simulink model "PositionObserver"  (R2020b)
settings: Solver=FixedStepDiscrete  StartTime=0.0  StopTime=100  RelTol=1e-3
values from neighbouring files (symbols this model uses):
  Ki_Iab_EMFobs = 1600.0    [MotorControl.sldd]
  Kp_Iab_EMFobs = 0.255    [MotorControl.sldd]
  Ts = 250.0e-06    (= 0.00025)    [MotorControlLibData.m]    (also in local_pmsm_torque_control_data.m = 5e-06)
undefined symbols (not defined in the file or in its folder): CuttOffFreq_c, EMFobsLdGain, EMFobsRS, MaxBckEMFVol_sat_neg, MaxBckEMFVol_sat_pos, TsIntern
libraries: pid_lib x2
settings Model: DataDictionary=MotorControl.sldd  Creator=unix  LastModifiedBy=unix
settings SolverCC: AutoInsertRateTranBlk=on
settings DataIOCC: SaveOutput=off  SaveTime=off
settings OptimizationCC: DefaultParameterBehavior=Inlined  EnhancedBackFolding=on  PassReuseOutputArgsAs=Individual arguments  ZeroExternalMemoryAtStartup=off  ZeroInternalMemoryAtStartup=off  OptimizeBlockOrder=speed  DifferentSizesBufferReuse=on  OptimizationCustomize=off  EfficientTunableParamExpr=on
settings DebuggingCC: SignalInfNanChecking=warning  SignalRangeChecking=warning  CheckMatrixSingularityMsg=warning  IntegerOverflowMsg=error  ParameterOverflowMsg=warning  ParameterUnderflowMsg=warning  ParameterPrecisionLossMsg=none  ParameterTunabilityLossMsg=error  UnderSpecifiedDataTypeMsg=warning  IntegerSaturationMsg=error
settings ModelReferenceCC: ModelReferenceNumInstancesAllowed=Single
settings SFSimCC: MATLABDynamicMemAlloc=off
settings RTWCC: Description=Embedded Coder  SystemTargetFile=ert.tlc  GenCodeOnly=on  TemplateMakefile=ert_default_tmf  GenerateReport=on  IncludeHyperlinkInReport=on  LaunchReport=on  GenerateTraceInfo=on  GenerateTraceReport=on  GenerateTraceReportSl=on  GenerateTraceReportSf=on  GenerateTraceReportEml=on
settings CodeAppCC: ForceParamTrailComments=on  IgnoreCustomStorageClasses=off  OperatorAnnotations=on  SimulinkDataObjDesc=on  SFDataObjDesc=on  InsertBlockDesc=on
settings ERTTargetCC: TargetLangStandard=C99 (ISO)  GenerateSampleERTMain=on  GenerateASAP2=on  InlinedParameterPlacement=NonHierarchical  ERTCustomFileTemplate=example_file_process.tlc

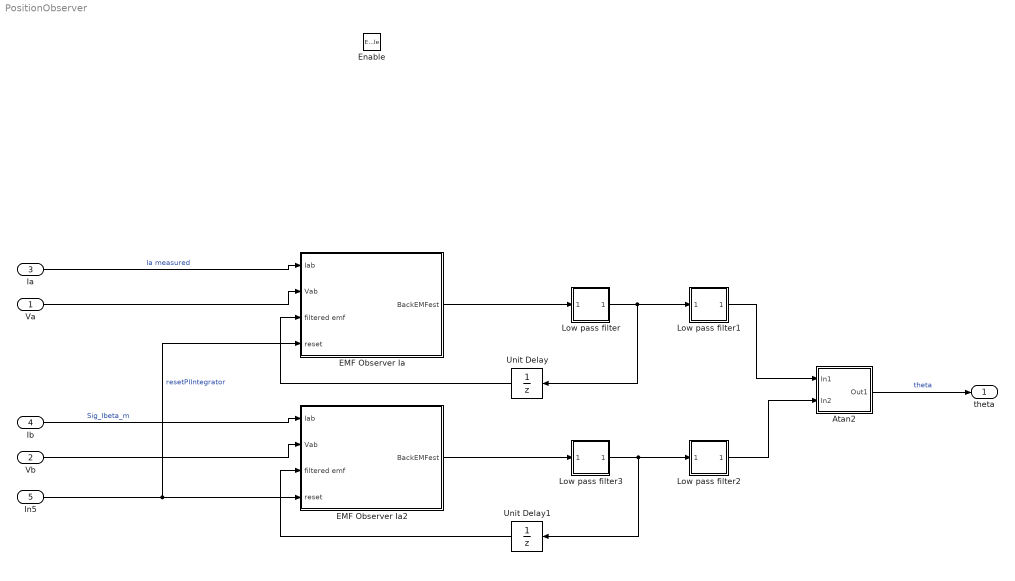
== system PositionObserver ==
  Va : Inport  OutDataTypeStr=fixdt(1,16,8)  PortDimensions=1  SampleTime=[0.00025000000000000001,0]
  Vb : Inport  Port=2  OutDataTypeStr=fixdt(1,16,8)  PortDimensions=1  SampleTime=[0.00025000000000000001,0]
  Ia : Inport  Port=3  OutDataTypeStr=fixdt(1,16,8)  PortDimensions=1  SampleTime=[0.00025000000000000001,0]
  Ib : Inport  Port=4  OutDataTypeStr=fixdt(1,16,8)  PortDimensions=1  SampleTime=[0.00025000000000000001,0]
  In5 : Inport  Port=5  OutDataTypeStr=boolean  PortDimensions=1  SampleTime=[0.00025000000000000001,0]
  Enable : EnablePort  StatesWhenEnabling=reset  SampleTime=[0.00025000000000000001,0]  OutDataTypeStr=boolean
  Atan2 : Subsystem
  EMF Observer Ia : Subsystem  mask{Rs=EMFobsRS, Ld=EMFobsLdGain, P=Kp_Iab_EMFobs, I=Ki_Iab_EMFobs}
      mask prompts: Rs "Resistance"; Ld "Inductance"; P "Simulink:masks:ProportionalP_MP"; I "Simulink:masks:IntegralI_MP"
      mask TypeOptions Rs: DC Motor Model/Resistance/Gain
      mask TypeOptions Ld: DC Motor Model/Inductance/Gain
      mask TypeOptions P: PID Controller/P
      mask TypeOptions I: PID Controller/I
      mask DialogControl Container6 Prompt: PI Controller
      mask DialogControl P Prompt: Proportional (P):
      mask DialogControl I Prompt: Integral (I):
  EMF Observer Ia2 : Subsystem  mask{Rs=EMFobsRS, Ld=EMFobsLdGain, P=Kp_Iab_EMFobs, I=Ki_Iab_EMFobs}
      mask prompts: Rs "Resistance"; Ld "Inductance"; P "Simulink:masks:ProportionalP_MP"; I "Simulink:masks:IntegralI_MP"
      mask TypeOptions Rs: DC Motor Model/Resistance/Gain
      mask TypeOptions Ld: DC Motor Model/Inductance/Gain
      mask TypeOptions P: PID Controller/P
      mask TypeOptions I: PID Controller/I
      mask DialogControl Container6 Prompt: PI Controller
      mask DialogControl P Prompt: Proportional (P):
      mask DialogControl I Prompt: Integral (I):
  Low pass filter : Subsystem  mask{Value=CuttOffFreq_c, Gain=250e-6}
      mask prompts: Value "CuttOff Freq."; Gain "Time interval"
      settings: AttributesFormatString=Integration constant %<Gain>
      mask TypeOptions Value: Constant/Value
      mask TypeOptions Gain: Gain/Gain
  Low pass filter1 : Subsystem  mask{Value=CuttOffFreq_c, Gain=250e-6}
      mask prompts: Value "CuttOff Freq."; Gain "Time interval"
      settings: AttributesFormatString=Integration constant %<Gain>
      mask TypeOptions Value: Constant/Value
      mask TypeOptions Gain: Gain/Gain
  Low pass filter2 : Subsystem  mask{Value=CuttOffFreq_c, Gain=250e-6}
      mask prompts: Value "CuttOff Freq."; Gain "Time interval"
      settings: AttributesFormatString=Integration constant %<Gain>
      mask TypeOptions Value: Constant/Value
      mask TypeOptions Gain: Gain/Gain
  Low pass filter3 : Subsystem  mask{Value=CuttOffFreq_c, Gain=250e-6}
      mask prompts: Value "CuttOff Freq."; Gain "Time interval"
      settings: AttributesFormatString=Integration constant %<Gain>
      mask TypeOptions Value: Constant/Value
      mask TypeOptions Gain: Gain/Gain
  Unit Delay : UnitDelay  SampleTime=-1  HasFrameUpgradeWarning=on
  Unit Delay1 : UnitDelay  SampleTime=-1  HasFrameUpgradeWarning=on
  theta : Outport  OutDataTypeStr=fixdt(1,16,8)  PortDimensions=1  SampleTime=[0.00025000000000000001,0]
  wires:
  Atan2/1(Out1) -> theta/1  "theta"
  Va/1 -> EMF Observer Ia/2(Vab)
  Ia/1 -> EMF Observer Ia/1(Iab)  "Ia measured"
  Vb/1 -> EMF Observer Ia2/2(Vab)
  Ib/1 -> EMF Observer Ia2/1(Iab)  "Sig_Ibeta_m"
  EMF Observer Ia/1(BackEMFest) -> Low pass filter/1(In1)
  Low pass filter/1(Output) -> Unit Delay/1, Low pass filter1/1(In1)
  EMF Observer Ia2/1(BackEMFest) -> Low pass filter3/1(In1)
  Low pass filter3/1(Output) -> Unit Delay1/1, Low pass filter2/1(In1)
  Low pass filter1/1(Output) -> Atan2/1(In1)
  Low pass filter2/1(Output) -> Atan2/2(In2)
  Unit Delay/1 -> EMF Observer Ia/3(filtered emf)
  Unit Delay1/1 -> EMF Observer Ia2/3(filtered emf)
  In5/1 -> EMF Observer Ia2/4(reset), EMF Observer Ia/4(reset)  "resetPIIntegrator"

== system PositionObserver/Atan2 ==
  In1 : Inport
  In2 : Inport  Port=2
  Atan2 : Trigonometry  Operator=atan2  ApproximationMethod=CORDIC  NumberOfIterations=6
  Data Type Conversion5 : DataTypeConversion
  Data Type Conversion6 : DataTypeConversion  OutDataTypeStr=single
  Data Type Conversion7 : DataTypeConversion  OutDataTypeStr=single
  Out1 : Outport
  wires:
  Data Type Conversion5/1 -> Out1/1
  In2/1 -> Data Type Conversion7/1
  Data Type Conversion7/1 -> Atan2/2
  Data Type Conversion6/1 -> Atan2/1
  In1/1 -> Data Type Conversion6/1
  Atan2/1 -> Data Type Conversion5/1

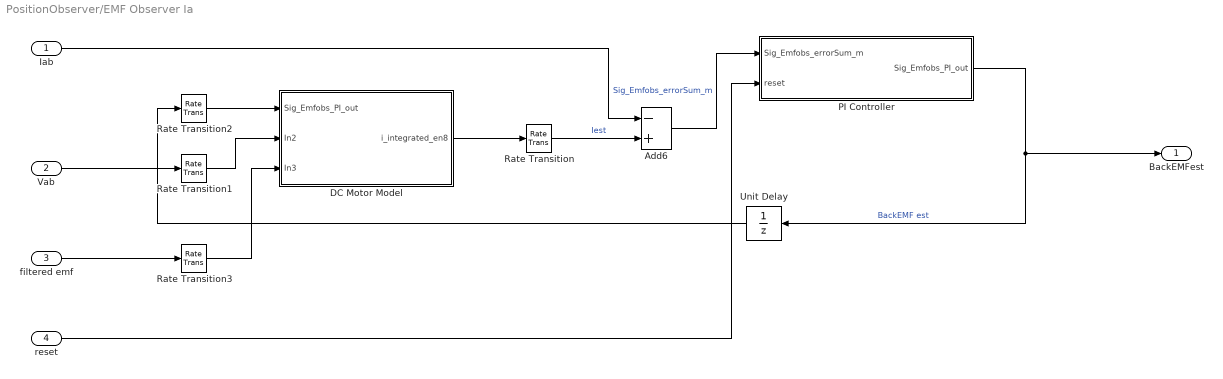
== system PositionObserver/EMF Observer Ia ==
  Iab : Inport
  Vab : Inport  Port=2
  filtered emf : Inport  Port=3
  reset : Inport  Port=4
  Add6 : Sum  Inputs=-+  InputSameDT=on
  DC Motor Model : Subsystem  TreatAsAtomicUnit=on  SystemSampleTime=Ts
  PI Controller : Subsystem
  Rate Transition{,1..3} (4 alike) : RateTransition  Integrity=off
  Unit Delay : UnitDelay  SampleTime=-1  HasFrameUpgradeWarning=on
  BackEMFest : Outport
  wires:
  reset/1 -> PI Controller/2(reset)
  Unit Delay/1 -> Rate Transition2/1
  Rate Transition3/1 -> DC Motor Model/3(In3)
  filtered emf/1 -> Rate Transition3/1
  Add6/1 -> PI Controller/1(Sig_Emfobs_errorSum_m)  "Sig_Emfobs_errorSum_m"
  PI Controller/1(Sig_Emfobs_PI_out) -> BackEMFest/1, Unit Delay/1  "BackEMF est"
  Rate Transition2/1 -> DC Motor Model/1(Sig_Emfobs_PI_out)
  Rate Transition1/1 -> DC Motor Model/2(In2)
  Rate Transition/1 -> Add6/2  "Iest"
  Vab/1 -> Rate Transition1/1
  DC Motor Model/1(i_integrated_en8) -> Rate Transition/1
  Iab/1 -> Add6/1

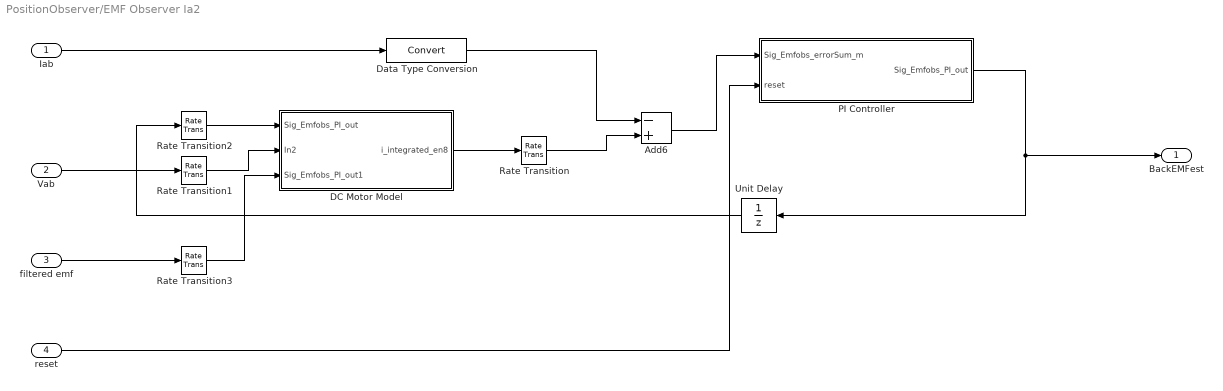
== system PositionObserver/EMF Observer Ia2 ==
  Iab : Inport
  Vab : Inport  Port=2
  filtered emf : Inport  Port=3
  reset : Inport  Port=4
  Add6 : Sum  Inputs=-+  InputSameDT=on
  DC Motor Model : Subsystem  TreatAsAtomicUnit=on  SystemSampleTime=Ts
  Data Type Conversion : DataTypeConversion
  PI Controller : Subsystem  TreatAsAtomicUnit=on
  Rate Transition{,1..3} (4 alike) : RateTransition  Integrity=off
  Unit Delay : UnitDelay  SampleTime=-1  HasFrameUpgradeWarning=on
  BackEMFest : Outport
  wires:
  reset/1 -> PI Controller/2(reset)
  Unit Delay/1 -> Rate Transition2/1
  Rate Transition3/1 -> DC Motor Model/3(Sig_Emfobs_PI_out1)
  filtered emf/1 -> Rate Transition3/1
  Data Type Conversion/1 -> Add6/1
  Iab/1 -> Data Type Conversion/1
  DC Motor Model/1(i_integrated_en8) -> Rate Transition/1
  Vab/1 -> Rate Transition1/1
  Rate Transition/1 -> Add6/2
  Rate Transition1/1 -> DC Motor Model/2(In2)
  Rate Transition2/1 -> DC Motor Model/1(Sig_Emfobs_PI_out)
  Add6/1 -> PI Controller/1(Sig_Emfobs_errorSum_m)
  PI Controller/1(Sig_Emfobs_PI_out) -> BackEMFest/1, Unit Delay/1

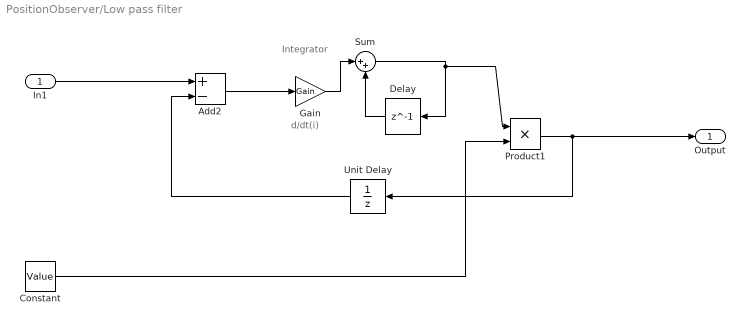
== system PositionObserver/Low pass filter ==
  note: d/dt(i)
  note: Integrator
  In1 : Inport
  Add2 : Sum  Inputs=+-
  Constant : Constant  Value=Value  OutDataTypeStr=fixdt(1,16,2^-15,0)
  Delay : Delay  DelayLength=1  InitialCondition=0
  Gain : Gain  Gain=Gain  ParamDataTypeStr=fixdt(1,16,2^-15,0)  OutMin=-100  OutMax=+100  OutDataTypeStr=fixdt(1,16,2^-4,0)  SaturateOnIntegerOverflow=on
  Product1 : Product  OutDataTypeStr=Inherit: Same as first input
  Sum : Sum  Inputs=|++  OutDataTypeStr=Inherit: Same as first input
  Unit Delay : UnitDelay  SampleTime=-1  HasFrameUpgradeWarning=on
  Output : Outport
  wires:
  Unit Delay/1 -> Add2/2
  Sum/1 -> Product1/1, Delay/1
  Delay/1 -> Sum/2
  Gain/1 -> Sum/1
  Product1/1 -> Unit Delay/1, Output/1
  Add2/1 -> Gain/1
  In1/1 -> Add2/1
  Constant/1 -> Product1/2

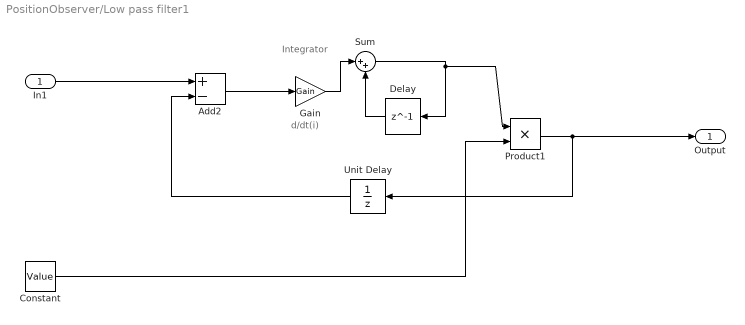
== system PositionObserver/Low pass filter1 ==
  note: Integrator
  note: d/dt(i)
  In1 : Inport
  Add2 : Sum  Inputs=+-
  Constant : Constant  Value=Value  OutDataTypeStr=fixdt(1,16,2^-15,0)
  Delay : Delay  DelayLength=1  InitialCondition=0
  Gain : Gain  Gain=Gain  ParamDataTypeStr=fixdt(1,16,2^-15,0)  OutMin=-100  OutMax=+100  OutDataTypeStr=fixdt(1,16,2^-4,0)  SaturateOnIntegerOverflow=on
  Product1 : Product  OutDataTypeStr=Inherit: Same as first input
  Sum : Sum  Inputs=|++  OutDataTypeStr=Inherit: Same as first input
  Unit Delay : UnitDelay  SampleTime=-1  HasFrameUpgradeWarning=on
  Output : Outport
  wires:
  Constant/1 -> Product1/2
  In1/1 -> Add2/1
  Add2/1 -> Gain/1
  Product1/1 -> Output/1, Unit Delay/1
  Gain/1 -> Sum/1
  Delay/1 -> Sum/2
  Sum/1 -> Delay/1, Product1/1
  Unit Delay/1 -> Add2/2

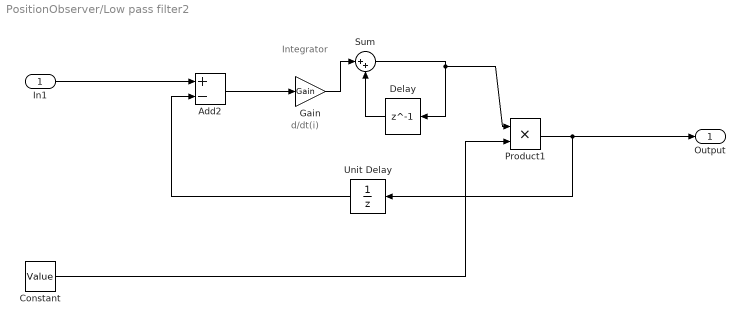
== system PositionObserver/Low pass filter2 ==
  note: d/dt(i)
  note: Integrator
  In1 : Inport
  Add2 : Sum  Inputs=+-
  Constant : Constant  Value=Value  OutDataTypeStr=fixdt(1,16,2^-15,0)
  Delay : Delay  DelayLength=1  InitialCondition=0
  Gain : Gain  Gain=Gain  ParamDataTypeStr=fixdt(1,16,2^-15,0)  OutMin=-100  OutMax=+100  OutDataTypeStr=fixdt(1,16,2^-4,0)  SaturateOnIntegerOverflow=on
  Product1 : Product  OutDataTypeStr=Inherit: Same as first input
  Sum : Sum  Inputs=|++  OutDataTypeStr=Inherit: Same as first input
  Unit Delay : UnitDelay  SampleTime=-1  HasFrameUpgradeWarning=on
  Output : Outport
  wires:
  Unit Delay/1 -> Add2/2
  Sum/1 -> Product1/1, Delay/1
  Delay/1 -> Sum/2
  Gain/1 -> Sum/1
  Product1/1 -> Unit Delay/1, Output/1
  Add2/1 -> Gain/1
  In1/1 -> Add2/1
  Constant/1 -> Product1/2

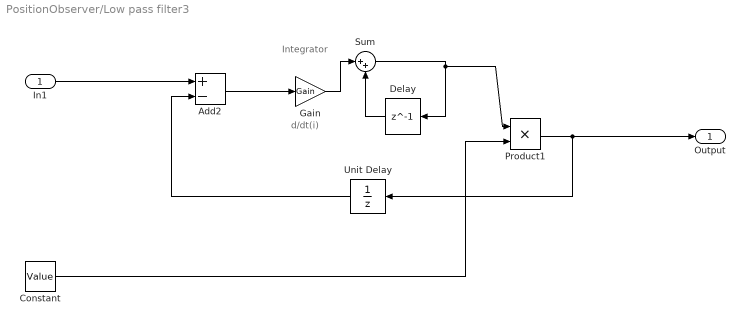
== system PositionObserver/Low pass filter3 ==
  note: Integrator
  note: d/dt(i)
  In1 : Inport
  Add2 : Sum  Inputs=+-
  Constant : Constant  Value=Value  OutDataTypeStr=fixdt(1,16,2^-15,0)
  Delay : Delay  DelayLength=1  InitialCondition=0
  Gain : Gain  Gain=Gain  ParamDataTypeStr=fixdt(1,16,2^-15,0)  OutMin=-100  OutMax=+100  OutDataTypeStr=fixdt(1,16,2^-4,0)  SaturateOnIntegerOverflow=on
  Product1 : Product  OutDataTypeStr=Inherit: Same as first input
  Sum : Sum  Inputs=|++  OutDataTypeStr=Inherit: Same as first input
  Unit Delay : UnitDelay  SampleTime=-1  HasFrameUpgradeWarning=on
  Output : Outport
  wires:
  Constant/1 -> Product1/2
  In1/1 -> Add2/1
  Add2/1 -> Gain/1
  Product1/1 -> Output/1, Unit Delay/1
  Gain/1 -> Sum/1
  Delay/1 -> Sum/2
  Sum/1 -> Delay/1, Product1/1
  Unit Delay/1 -> Add2/2

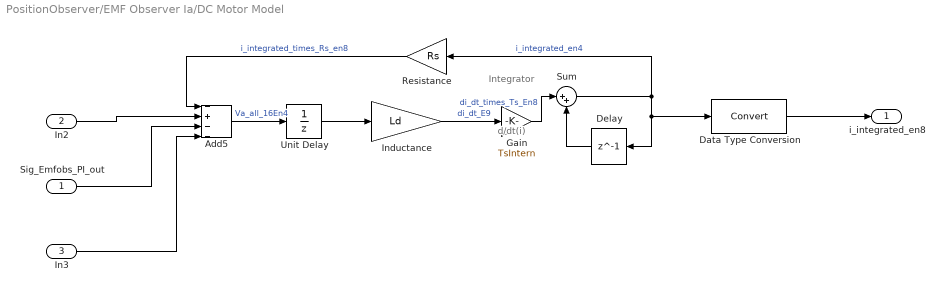
== system PositionObserver/EMF Observer Ia/DC Motor Model ==
  note: Integrator
  note: d/dt(i)
  Sig_Emfobs_PI_out : Inport
  In2 : Inport  Port=2
  In3 : Inport  Port=3
  Add5 : Sum  Inputs=-+--  OutDataTypeStr=Inherit: Same as first input
  Data Type Conversion : DataTypeConversion
  Delay : Delay  DelayLength=1  InitialCondition=0  StateName=UnitDelayIntegratorPosObs
  Gain : Gain  Gain=TsIntern  ParamDataTypeStr=Inherit: Inherit from 'Gain'  OutMin=-100  OutMax=+100  OutDataTypeStr=fixdt(1,16,2^-4,0)  SaturateOnIntegerOverflow=on
  Inductance : Gain  Gain=Ld  OutDataTypeStr=fixdt(1,16,2^9,0)
  Resistance : Gain  Gain=Rs  OutDataTypeStr=Inherit: Inherit via back propagation
  Sum : Sum  Inputs=|++  OutDataTypeStr=Inherit: Same as first input
  Unit Delay : UnitDelay  SampleTime=-1  HasFrameUpgradeWarning=on
  i_integrated_en8 : Outport
  wires:
  In3/1 -> Add5/4
  Data Type Conversion/1 -> i_integrated_en8/1
  Inductance/1 -> Gain/1  "di_dt_E9"
  Add5/1 -> Unit Delay/1  "Va_all_16En4"
  Sig_Emfobs_PI_out/1 -> Add5/3
  Delay/1 -> Sum/2
  Resistance/1 -> Add5/1  "i_integrated_times_Rs_en8"
  In2/1 -> Add5/2
  Sum/1 -> Resistance/1, Data Type Conversion/1, Delay/1  "i_integrated_en4"
  Gain/1 -> Sum/1  "di_dt_times_Ts_En8"
  Unit Delay/1 -> Inductance/1

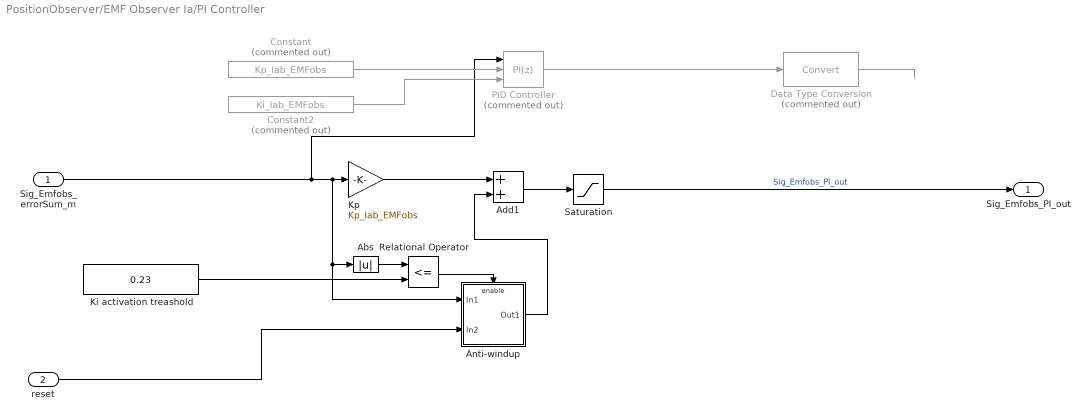
== system PositionObserver/EMF Observer Ia/PI Controller ==
  Sig_Emfobs_errorSum_m : Inport
  reset : Inport  Port=2
  Abs : Abs
  Add1 : Sum
  Anti-windup : Subsystem
  Constant : Constant  Commented=on  Value=Kp_Iab_EMFobs
  Constant2 : Constant  Commented=on  Value=Ki_Iab_EMFobs
  Data Type Conversion : DataTypeConversion  Commented=on
  Ki activation treashold : Constant  Value=0.23  OutDataTypeStr=fixdt(1,16,2^-8,0)
  Kp : Gain  Gain=Kp_Iab_EMFobs  OutDataTypeStr=Inherit: Same as input
  PID Controller : pid_lib/PID Controller  Commented=on  Controller=PI  Form=Parallel  TimeDomain=Discrete-time  UseExternalTs=off  SampleTime=-1  IntegratorMethod=Forward Euler  FilterMethod=Forward Euler  ControllerParametersSource=external  P=1  I=1  D=0  UseFilter=on  N=100  TunerSelectOption=Transfer Function Based (PID Tuner App)  ZeroCross=off  InitialConditionSource=internal  InitialConditionForIntegrator=0  InitialConditionForFilter=0  DifferentiatorICPrevScaledInput=0  ExternalReset=none  TrackingMode=off  Kt=1  LimitOutput=on  SatLimitsSource=internal  UpperSaturationLimit=MaxBckEMFVol_sat_pos  LowerSaturationLimit=MaxBckEMFVol_sat_neg  LinearizeAsGain=on  AntiWindupMode=clamping  Kb=1  POutMin=[]  POutMax=[]  IOutMin=[]  IOutMax=[]  DOutMin=[]  DOutMax=[]  NOutMin=[]  NOutMax=[]  SumOutMin=[]  SumOutMax=[]  SaturationOutMin=[]  SaturationOutMax=[]  PParamMin=[]  PParamMax=[]  IParamMin=[]  IParamMax=[]  DParamMin=[]  DParamMax=[]  NParamMin=[]  NParamMax=[]  KbParamMin=[]  KbParamMax=[]  KtParamMin=[]  KtParamMax=[]  KbOutMin=[]  KbOutMax=[]  KtOutMin=[]  KtOutMax=[]  IntegratorOutMin=[]  IntegratorOutMax=[]  FilterOutMin=[]  FilterOutMax=[]  SumI1OutMin=[]  SumI1OutMax=[]  SumI2OutMin=[]  SumI2OutMax=[]  SumI3OutMin=[]  SumI3OutMax=[]  SumI4OutMin=[]  SumI4OutMax=[]  SumDOutMin=[]  SumDOutMax=[]  DifferentiatorOutMin=[]  DifferentiatorOutMax=[]  FilterDiffOutCoefMin=[]  FilterDiffOutCoefMax=[]  ReciprocalOutMin=[]  ReciprocalOutMax=[]  SumDenOutMin=[]  SumDenOutMax=[]  SumNumOutMin=[]  SumNumOutMax=[]  DivideOutMin=[]  DivideOutMax=[]  UdiffTsProdOutMin=[]  UdiffTsProdOutMax=[]  NTsProdOutMin=[]  NTsProdOutMax=[]  UintegralTsProdOutMin=[]  UintegralTsProdOutMax=[]  UngainTsProdOutMin=[]  UngainTsProdOutMax=[]  IntegratorContinuousStateAttributes=''  IntegratorStateMustResolveToSignalObject=off  IntegratorRTWStateStorageClass=Auto  FilterContinuousStateAttributes=''  FilterStateMustResolveToSignalObject=off  FilterRTWStateStorageClass=Auto  ParallelPVariant=ExternalParameters  IdealPVariant=Disabled  IVariant=ExternalParameters  DVariant=Disabled  IntegratorVariant=Discrete  SatVariant=Enabled  AWVariant=DiscClampingParallel  PCopyVariant=Disabled  TRVariant=Disabled  FdbkBlocksVariant=Forward  IdealPFdbkVariant=Disabled  SatFdbkVariant=Disabled  DerivativeFilterVariant=Disabled  NVariant=Disabled  NCopyVariant=Disabled_SignalSpec  FilterICVariant=Disabled  IntegratorICVariant=InternalICs  ExternalResetVariant=Disabled  TRSumVariant=Passthrough  SumFdbkVariant=Disabled  SumVariant=Sum_PI  TsampFilterVariant=InternalTs  TsampNgainVariant=Passthrough  TsampIntegralVariant=Passthrough  ExternalSaturationOutDataTypeStr=Inherit: Same as second input
  Relational Operator : RelationalOperator  Operator=<=  OutDataTypeStr=boolean  RndMeth=Simplest
  Saturation : Saturate  UpperLimit=MaxBckEMFVol_sat_pos  LowerLimit=MaxBckEMFVol_sat_neg
  Sig_Emfobs_PI_out : Outport
  wires:
  reset/1 -> Anti-windup/2(In2)
  Abs/1 -> Relational Operator/1
  Saturation/1 -> Sig_Emfobs_PI_out/1  "Sig_Emfobs_PI_out"
  Sig_Emfobs_errorSum_m/1 -> Kp/1, Abs/1, Anti-windup/1(In1), PID Controller/1
  Data Type Conversion/1 -> ?
  Constant2/1 -> PID Controller/3
  Constant/1 -> PID Controller/2
  Relational Operator/1 -> Anti-windup/Enable
  Add1/1 -> Saturation/1
  Ki activation treashold/1 -> Relational Operator/2
  Anti-windup/1(Out1) -> Add1/2
  Kp/1 -> Add1/1
  PID Controller/1 -> Data Type Conversion/1

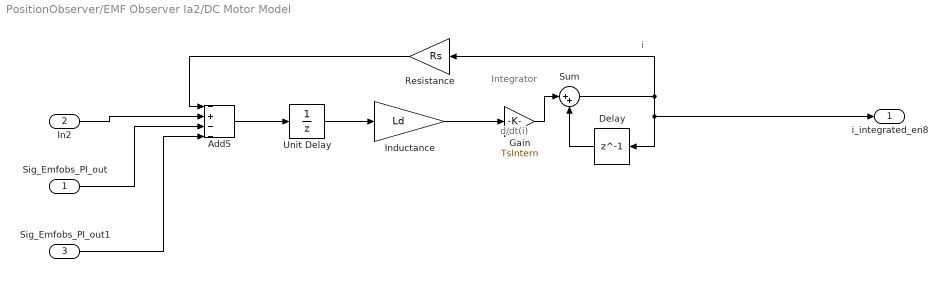
== system PositionObserver/EMF Observer Ia2/DC Motor Model ==
  note: i
  note: d/dt(i)
  note: Integrator
  Sig_Emfobs_PI_out : Inport
  In2 : Inport  Port=2
  Sig_Emfobs_PI_out1 : Inport  Port=3
  Add5 : Sum  Inputs=-+--  OutDataTypeStr=Inherit: Same as first input
  Delay : Delay  DelayLength=1  InitialCondition=0
  Gain : Gain  Gain=TsIntern  ParamDataTypeStr=Inherit: Inherit from 'Gain'  OutMin=-100  OutMax=+100  OutDataTypeStr=fixdt(1,16,2^-4,0)  SaturateOnIntegerOverflow=on
  Inductance : Gain  Gain=Ld  OutDataTypeStr=fixdt(1,16,2^9,0)
  Resistance : Gain  Gain=Rs  OutDataTypeStr=Inherit: Inherit via back propagation
  Sum : Sum  Inputs=|++  OutDataTypeStr=Inherit: Same as first input
  Unit Delay : UnitDelay  SampleTime=-1  HasFrameUpgradeWarning=on
  i_integrated_en8 : Outport
  wires:
  Sig_Emfobs_PI_out1/1 -> Add5/4
  Unit Delay/1 -> Inductance/1
  Gain/1 -> Sum/1
  In2/1 -> Add5/2
  Resistance/1 -> Add5/1
  Delay/1 -> Sum/2
  Sig_Emfobs_PI_out/1 -> Add5/3
  Add5/1 -> Unit Delay/1
  Inductance/1 -> Gain/1
  Sum/1 -> Delay/1, i_integrated_en8/1, Resistance/1

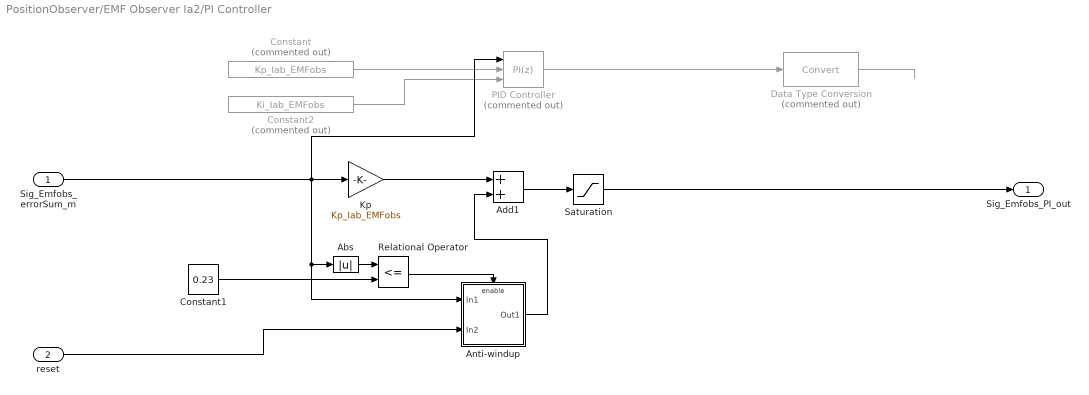
== system PositionObserver/EMF Observer Ia2/PI Controller ==
  Sig_Emfobs_errorSum_m : Inport
  reset : Inport  Port=2
  Abs : Abs
  Add1 : Sum
  Anti-windup : Subsystem
  Constant : Constant  Commented=on  Value=Kp_Iab_EMFobs
  Constant1 : Constant  Value=0.23  OutDataTypeStr=fixdt(1,16,2^-8,0)
  Constant2 : Constant  Commented=on  Value=Ki_Iab_EMFobs
  Data Type Conversion : DataTypeConversion  Commented=on
  Kp : Gain  Gain=Kp_Iab_EMFobs  ParamDataTypeStr=Inherit: Inherit from 'Gain'  OutDataTypeStr=Inherit: Same as input
  PID Controller : pid_lib/PID Controller  Commented=on  Controller=PI  Form=Parallel  TimeDomain=Discrete-time  UseExternalTs=off  SampleTime=-1  IntegratorMethod=Forward Euler  FilterMethod=Forward Euler  ControllerParametersSource=external  P=1  I=1  D=0  UseFilter=on  N=100  TunerSelectOption=Transfer Function Based (PID Tuner App)  ZeroCross=off  InitialConditionSource=internal  InitialConditionForIntegrator=0  InitialConditionForFilter=0  DifferentiatorICPrevScaledInput=0  ExternalReset=none  TrackingMode=off  Kt=1  LimitOutput=on  SatLimitsSource=internal  UpperSaturationLimit=MaxBckEMFVol_sat_pos  LowerSaturationLimit=MaxBckEMFVol_sat_neg  LinearizeAsGain=on  AntiWindupMode=clamping  Kb=1  POutMin=[]  POutMax=[]  IOutMin=[]  IOutMax=[]  DOutMin=[]  DOutMax=[]  NOutMin=[]  NOutMax=[]  SumOutMin=[]  SumOutMax=[]  SaturationOutMin=[]  SaturationOutMax=[]  PParamMin=[]  PParamMax=[]  IParamMin=[]  IParamMax=[]  DParamMin=[]  DParamMax=[]  NParamMin=[]  NParamMax=[]  KbParamMin=[]  KbParamMax=[]  KtParamMin=[]  KtParamMax=[]  KbOutMin=[]  KbOutMax=[]  KtOutMin=[]  KtOutMax=[]  IntegratorOutMin=[]  IntegratorOutMax=[]  FilterOutMin=[]  FilterOutMax=[]  SumI1OutMin=[]  SumI1OutMax=[]  SumI2OutMin=[]  SumI2OutMax=[]  SumI3OutMin=[]  SumI3OutMax=[]  SumI4OutMin=[]  SumI4OutMax=[]  SumDOutMin=[]  SumDOutMax=[]  DifferentiatorOutMin=[]  DifferentiatorOutMax=[]  FilterDiffOutCoefMin=[]  FilterDiffOutCoefMax=[]  ReciprocalOutMin=[]  ReciprocalOutMax=[]  SumDenOutMin=[]  SumDenOutMax=[]  SumNumOutMin=[]  SumNumOutMax=[]  DivideOutMin=[]  DivideOutMax=[]  UdiffTsProdOutMin=[]  UdiffTsProdOutMax=[]  NTsProdOutMin=[]  NTsProdOutMax=[]  UintegralTsProdOutMin=[]  UintegralTsProdOutMax=[]  UngainTsProdOutMin=[]  UngainTsProdOutMax=[]  IntegratorContinuousStateAttributes=''  IntegratorStateMustResolveToSignalObject=off  IntegratorRTWStateStorageClass=Auto  FilterContinuousStateAttributes=''  FilterStateMustResolveToSignalObject=off  FilterRTWStateStorageClass=Auto  ParallelPVariant=ExternalParameters  IdealPVariant=Disabled  IVariant=ExternalParameters  DVariant=Disabled  IntegratorVariant=Discrete  SatVariant=Enabled  AWVariant=DiscClampingParallel  PCopyVariant=Disabled  TRVariant=Disabled  FdbkBlocksVariant=Forward  IdealPFdbkVariant=Disabled  SatFdbkVariant=Disabled  DerivativeFilterVariant=Disabled  NVariant=Disabled  NCopyVariant=Disabled_SignalSpec  FilterICVariant=Disabled  IntegratorICVariant=InternalICs  ExternalResetVariant=Disabled  TRSumVariant=Passthrough  SumFdbkVariant=Disabled  SumVariant=Sum_PI  TsampFilterVariant=InternalTs  TsampNgainVariant=Passthrough  TsampIntegralVariant=Passthrough  ExternalSaturationOutDataTypeStr=Inherit: Same as second input
  Relational Operator : RelationalOperator  Operator=<=  OutDataTypeStr=boolean  RndMeth=Simplest
  Saturation : Saturate  UpperLimit=MaxBckEMFVol_sat_pos  LowerLimit=MaxBckEMFVol_sat_neg
  Sig_Emfobs_PI_out : Outport
  wires:
  reset/1 -> Anti-windup/2(In2)
  Abs/1 -> Relational Operator/1
  PID Controller/1 -> Data Type Conversion/1
  Kp/1 -> Add1/1
  Anti-windup/1(Out1) -> Add1/2
  Constant1/1 -> Relational Operator/2
  Add1/1 -> Saturation/1
  Relational Operator/1 -> Anti-windup/Enable
  Constant/1 -> PID Controller/2
  Constant2/1 -> PID Controller/3
  Data Type Conversion/1 -> ?
  Sig_Emfobs_errorSum_m/1 -> PID Controller/1, Abs/1, Anti-windup/1(In1), Kp/1
  Saturation/1 -> Sig_Emfobs_PI_out/1

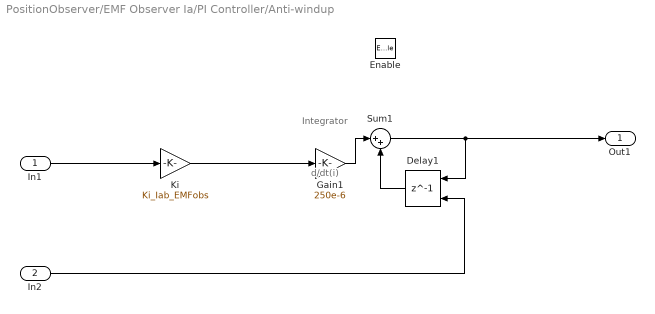
== system PositionObserver/EMF Observer Ia/PI Controller/Anti-windup ==
  note: Integrator
  note: d/dt(i)
  In1 : Inport
  In2 : Inport  Port=2
  Enable : EnablePort
  Delay1 : Delay  DelayLength=1  InitialCondition=0  ExternalReset=Level
      settings: InputPortMap=u0,r5
  Gain1 : Gain  Gain=250e-6  ParamDataTypeStr=fixdt(1,16,2^-16,0)  OutDataTypeStr=fixdt(1,16,2^-12,0)
  Ki : Gain  Gain=Ki_Iab_EMFobs  ParamDataTypeStr=Inherit: Inherit from 'Gain'  OutDataTypeStr=Inherit: Same as input
  Sum1 : Sum  Inputs=|++  OutDataTypeStr=fixdt(1,16,2^-8,0)
  Out1 : Outport
  wires:
  In2/1 -> Delay1/2
  Ki/1 -> Gain1/1
  In1/1 -> Ki/1
  Delay1/1 -> Sum1/2
  Gain1/1 -> Sum1/1
  Sum1/1 -> Delay1/1, Out1/1

== system PositionObserver/EMF Observer Ia2/PI Controller/Anti-windup ==
  note: d/dt(i)
  note: Integrator
  In1 : Inport
  In2 : Inport  Port=2
  Enable : EnablePort
  Delay1 : Delay  DelayLength=1  InitialCondition=0  ExternalReset=Level
      settings: InputPortMap=u0,r5
  Gain1 : Gain  Gain=250e-6  ParamDataTypeStr=fixdt(1,16,2^-16,0)  OutDataTypeStr=fixdt(1,16,2^-12,0)
  Ki : Gain  Gain=Ki_Iab_EMFobs  ParamDataTypeStr=Inherit: Inherit from 'Gain'  OutDataTypeStr=Inherit: Same as input
      settings: AttributesFormatString=%<Gain>
  Sum1 : Sum  Inputs=|++  OutDataTypeStr=fixdt(1,16,2^-8,0)
  Out1 : Outport
  wires:
  In2/1 -> Delay1/2
  Sum1/1 -> Out1/1, Delay1/1
  Gain1/1 -> Sum1/1
  Delay1/1 -> Sum1/2
  In1/1 -> Ki/1
  Ki/1 -> Gain1/1
